simulink model "mirageTracking"  (R2015a)
settings: Solver=FixedStepDiscrete  StartTime=0.0  StopTime=10  FixedStep=1/30  RelTol=1e-3
undefined symbols (not defined in the file or in its folder): IsPositionTracked, IsSkeletonTracked, JointDepthIndices, JointImageIndices, JointTrackingState, JointWorldCoordinates, none, PositionDepthIndices, PositionImageIndices, PositionWorldCoordinates, SegmentationData, SkeletonTrackingID, videoinput
libraries: imaqlib x2
settings Model: xpc_rtwmakecfg_data=_jpeg_  CovSFcnEnable=off  Creator=sd0016  LastModifiedBy=sd0016
settings DebuggingCC: SolverPrmCheckMsg=warning
settings RTWCC: BuildConfiguration=Faster Runs

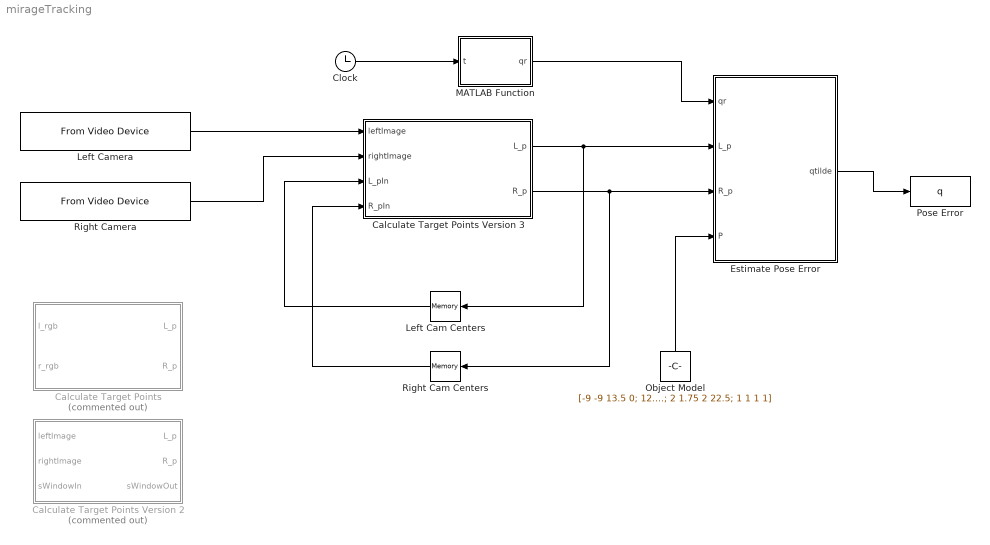
== system mirageTracking ==
  Calculate Target Points : MATLAB Function  Commented=on  TreatAsAtomicUnit=on
  Calculate Target Points Version 2 : MATLAB Function  Commented=on  TreatAsAtomicUnit=on
  Calculate Target Points Version 3 : MATLAB Function  TreatAsAtomicUnit=on
  Clock : Clock
  Estimate Pose Error : MATLAB Function  TreatAsAtomicUnit=on
  Left Cam Centers : Memory  X0=[598.500000000000,692.500000000000,645.500000000000,645.045454545455;681.157142857143,682.500000000000,673.159090909091,602.681818181818]  InheritSampleTime=on
  Left Camera : imaqlib/From Video Device  DeviceMenu=(none)  Device=winvideo 1 (Logitech HD Webcam C525)  ObjConstructor=videoinput('winvideo', 1)  VideoFormatMenu=(none)  VideoFormat=RGB24_1280x960  VideoSource=input1  ROIPosition=[0 0 960 1280]  EnableHWTrigger=off  TriggerConfiguration=none/none  SampleTime=1/30  OutputPortsMode=One multidimensional signal  DataType=single  CanDoHWTrigger=no  ReturnedColorSpace=rgb  BlockHandle=1921.0006  ROIWidth=1280  ROIHeight=960  ROIColumn=0  ROIRow=0  EngXMLPath=C:\Program Files\MATLAB\R2015a\toolbox\imaq\imaq\private  DevXMLPath=C:\MATLAB\SupportPackages\R2015a\osgenericvideointerface\toolbox\imaq\supportpackages\genericvideo\adaptor\win64  EngLibPath=C:\Program Files\MATLAB\R2015a\toolbox\imaq\imaqblks\imaqmex\win64  ColorSpace=rgb  BayerSensorAlignment=grbg  AllMetadata=IsPositionTracked;IsSkeletonTracked;JointDepthIndices;JointImageIndices;JointTrackingState;JointWorldCoordinates;PositionDepthIndices;PositionImageIndices;PositionWorldCoordinates;SegmentationData;SkeletonTrackingID
  MATLAB Function : MATLAB Function  TreatAsAtomicUnit=on
  Object Model : Constant  Value=[-9 -9 13.5 0; 12.75 -12.75 0 0; 2 1.75 2 22.5; 1 1 1 1]  VectorParams1D=off
  Pose Error : ToWorkspace  VariableName=q  SampleTime=-1
  Right Cam Centers : Memory  X0=[566.500000000000,660.814516129032,616.161764705882,612.663934426230;756.500000000000,756.250000000000,747.161764705882,676.614754098361]  InheritSampleTime=on
  Right Camera : imaqlib/From Video Device  DeviceMenu=(none)  Device=winvideo 2 (Logitech HD Webcam C525)  ObjConstructor=videoinput('winvideo', 2)  VideoFormatMenu=(none)  VideoFormat=RGB24_1280x960  VideoSource=input1  ROIPosition=[0 0 960 1280]  EnableHWTrigger=off  TriggerConfiguration=none/none  SampleTime=1/30  OutputPortsMode=One multidimensional signal  DataType=single  CanDoHWTrigger=no  ReturnedColorSpace=rgb  BlockHandle=1921.0006  ROIWidth=1280  ROIHeight=960  ROIColumn=0  ROIRow=0  EngXMLPath=C:\Program Files\MATLAB\R2015a\toolbox\imaq\imaq\private  DevXMLPath=C:\MATLAB\SupportPackages\R2015a\osgenericvideointerface\toolbox\imaq\supportpackages\genericvideo\adaptor\win64  EngLibPath=C:\Program Files\MATLAB\R2015a\toolbox\imaq\imaqblks\imaqmex\win64  ColorSpace=rgb  BayerSensorAlignment=grbg  AllMetadata=IsPositionTracked;IsSkeletonTracked;JointDepthIndices;JointImageIndices;JointTrackingState;JointWorldCoordinates;PositionDepthIndices;PositionImageIndices;PositionWorldCoordinates;SegmentationData;SkeletonTrackingID
  wires:
  Clock/1 -> MATLAB Function/1(t)
  MATLAB Function/1(qr) -> Estimate Pose Error/1(qr)
  Object Model/1 -> Estimate Pose Error/4(P)
  Estimate Pose Error/1(qtilde) -> Pose Error/1
  Left Camera/1 -> Calculate Target Points Version 3/1(leftImage)
  Right Camera/1 -> Calculate Target Points Version 3/2(rightImage)
  Calculate Target Points Version 3/1(L_p) -> Left Cam Centers/1, Estimate Pose Error/2(L_p)
  Calculate Target Points Version 3/2(R_p) -> Right Cam Centers/1, Estimate Pose Error/3(R_p)
  Left Cam Centers/1 -> Calculate Target Points Version 3/3(L_pIn)
  Right Cam Centers/1 -> Calculate Target Points Version 3/4(R_pIn)

== matlab function mirageTracking/Calculate Target Points ==
  data: l_rgb input; L_p output; r_rgb input; R_p output
function [L_p, R_p] = getCenter(l_rgb,r_rgb)

    %#codegen
    L_p=zeros(2,4);
    R_p=zeros(2,4);
    
    %input left image(l_rgb), right image(r_rgb), Pose target position 
    [m,n,c]=size(l_rgb);
    
    %define image variables for processing
    l_gray=zeros(m,n);      r_gray=zeros(m,n);
    l_rgb1=zeros(m,n,c);    r_rgb1=zeros(m,n,c);
    l_rgb2=zeros(m,n);      r_rgb2=zeros(m,n);

    l_bw=false(m,n);        r_bw=false(m,n);
    
    l_rgb1 = imcomplement(l_rgb);        % converts RGB to CMY color space 
    r_rgb1 = imcomplement(r_rgb);        % converts RGB to CMY color space 
    
    l_gray = 0.2989 * l_rgb1(:,:,1) + 0.5870 * l_rgb1(:,:,2) + 0.1140 * l_rgb1(:,:,3); % rgb2gray(rgb) ;convert rgb to grayscale 
    r_gray = 0.2989 * r_rgb1(:,:,1) + 0.5870 * r_rgb1(:,:,2) + 0.1140 * r_rgb1(:,:,3); % rgb2gray(rgb) ;convert rgb to grayscale
    
    l_rgb2 = l_rgb1(:,:,3)-l_gray;       % imsubtract(rgb1(:,:,3),gray)
    r_rgb2 = r_rgb1(:,:,3)-r_gray;       % imsubtract(rgb1(:,:,3),gray) 
        
%     l_rgb2 = medfilt2(l_rgb2);     % medfilt2(rgb2,[3 3]);
%     r_rgb2 = medfilt2(r_rgb2);     % medfilt2(rgb2,[3 3]);
%       
%     l_rgb2 = myMat2gray(l_rgb2);
%     r_rgb2 = myMat2gray(r_rgb2);
     
    l_bw = l_rgb2 > 0.2;
    r_bw = r_rgb2 > 0.2;

    %finds yellow regions in image using BlobAnalysis.
    hblob = vision.BlobAnalysis;

    [~,l_center,~] = step(hblob, l_bw); % get [x y] is a centroid of region
    [~,r_center,~] = step(hblob, r_bw); % get [x y] is a centroid of region
    
    %Send Left Camera Points
    ml = size(l_center,1);
    if ml > 4
        ml = 4;
    end
    
    for i=1:ml
        L_p(:,i)=l_center(i,:);
    end
    
    %Send Right Camera Points
    mr = size(r_center,1);
    if mr > 4
        mr = 4;
    end
    for i=1:mr
        R_p(:,i)=r_center(i,:);
    end
        
    L_p = orderPoints(L_p,m); 
    R_p = orderPoints(R_p,m);
        
    L_p(2,:) = m - L_p(2,:);
    R_p(2,:) = m - R_p(2,:);
end

% function imgOut = myMat2gray(imgIn)
%     %#codegen
%     imgIn = double(imgIn);
%     
%     minL = min(imgIn(:));
%     
%     imgTmp = (imgIn - minL);
%     
%     maxL = max(imgTmp(:));
%     
%     imgOut = imgTmp/maxL;
% end

== matlab function mirageTracking/MATLAB Function ==
  data: t input; qr output
function qr  = desired(t)
%#codegen

% qr = [xr yr thetar]^T (reference trajectory)
% ur = [vr omegar]^T (reference control input that generates the reference trajetory in ideal conditions)

% A = 1;
% xL = 10;
% vx = 1;

% % 
% % desired x and y 
% xr = vx*t;
% yr = A*sin(2*pi*xr/xL);
% 
% % desired x and y derivatives
% xrdot = vx;
% yrdot = A*(2*pi/xL)*cos(2*pi*xr/xL);
% 
% % desired theta
% thetar = atan2(yrdot,xrdot);
% 
% % desired second derivatives
% xrddot = 0;
% yrddot = -A*(2*pi/xL)^2*sin(2*pi*xr/xL);
% 
% % desired theta derivative
% thetardot = (yrddot - xrddot*tan(thetar))/(xrdot*(1+tan(thetar)^2));
% 
% 
% vr     = sqrt(xrdot^2+yrdot^2);
% omegar = thetardot;

%--------------------------------------------
% 
% xr = vx*t - 30;
% yr = A*sin(2*pi*xr/xL) + 2;
% 
% % desired x and y derivatives
% xrdot = vx;
% yrdot = A*(2*pi/xL)*cos(2*pi*xr/xL);
% 
% % desired theta
% thetar = atan2(yrdot,xrdot);
% 
% % desired second derivatives
% xrddot = 0;
% yrddot = -A*(2*pi/xL)^2*sin(2*pi*xr/xL);
% 
% % desired theta derivative
% thetardot = (yrddot - xrddot*tan(thetar))/(xrdot*(1+tan(thetar)^2));
% 
% vr     = sqrt(xrdot^2+yrdot^2);
% omegar = thetardot;

%--------------------------------------------
% yr = vx*t - 30;
% xr = A*sin(2*pi*yr/xL) + 2;
% 
% yrdot = vx;
% xrdot = A*(2*pi/xL)*cos(2*pi*xr/xL);
% 
% desired theta
% thetar = atan2(yrdot,xrdot);
% thetardot = 0;
% 
% vr     = sqrt(xrdot^2+yrdot^2);
% omegar = thetardot;

%--------------------------------------------
% xr = vx*t - 30;
% yr = 5;
% 
% xrdot = vx;
% yrdot = 0;
% 
% thetar = 0;
% thetardot = 0;
% 
% vr     = sqrt(xrdot^2+yrdot^2);
% omegar = thetardot;

% qr = [xr;yr;thetar];
% ur = [vr;omegar];

qr = [-395 2 45 0 0 0]';

== matlab function mirageTracking/Estimate Pose Error ==
  data: qr input; qtilde output; L_p input; R_p input; P input
function qtilde = mirage(qr,L_p,R_p,P)
%#codegen

%Desired Robot Pose for current step qr()
robotPoseDes.x = qr(1);
robotPoseDes.y = qr(2);
robotPoseDes.z = qr(3);
robotPoseDes.phi = qr(4);
robotPoseDes.theta = qr(5);
robotPoseDes.psi = qr(6);

%Transform target points from I space into Desired Robot Space
world2robotDes = inv(EulerTrans(robotPoseDes));
S_PDes = world2robotDes*P;

%Calculate the error parameters for current step
errParams = visioMotor(L_p,R_p,S_PDes);

poseErrorMat = eye(4,4);
poseErrorMat(1:3,:) = reshape(errParams,3,4);

world2robot = poseErrorMat*world2robotDes;

robotPoseEst = calculatePose(world2robot);

qtilde = [ -robotPoseEst.x  - robotPoseDes.x;
           -robotPoseEst.y  - robotPoseDes.y;
           -robotPoseEst.z  - robotPoseDes.z;
           -robotPoseEst.phi  - robotPoseDes.phi;
           -robotPoseEst.theta  - robotPoseDes.theta;
           -robotPoseEst.psi  - robotPoseDes.psi;];
       
end

== matlab function mirageTracking/Calculate Target Points Version 2 ==
  data: leftImage input; L_p output; rightImage input; sWindowIn input; R_p output; sWindowOut output
function [L_p, R_p, sWindowOut] = getCenterV2(leftImage, rightImage, sWindowIn)

    %#codegen
    L_p=zeros(2,4);
    R_p=zeros(2,4);
    
    m = size(leftImage,1);
    sWindowOut = zeros(8,4);
    
    for i=1:4
        lw = sWindowIn(i,:);
        lwx = (1:80) + lw(1);
        lwy = (1:80) + lw(2);
        
        rw = sWindowIn(i+4,:);
        rwx = (1:80) + rw(1);
        rwy = (1:80) + rw(2);
        
        pWinL = leftImage(lwy,lwx,:);
        pWinR = rightImage(rwy,rwx,:);
                
        pWinL = imcomplement(pWinL);        
        pWinR = imcomplement(pWinR);        
    
        pGrayL = 0.2989 * pWinL(:,:,1) + 0.5870 * pWinL(:,:,2) + 0.1140 * pWinL(:,:,3);
        pGrayR = 0.2989 * pWinR(:,:,1) + 0.5870 * pWinR(:,:,2) + 0.1140 * pWinR(:,:,3);
    
        pWinLF = pWinL(:,:,3)-pGrayL;       % imsubtract(rgb1(:,:,3),gray)
        pWinRF = pWinR(:,:,3)-pGrayR;       % imsubtract(rgb1(:,:,3),gray) 

        pBWL = pWinLF > 0.2;
        pBWR = pWinRF > 0.2;

        hblob = vision.BlobAnalysis; %finds yellow regions in image using BlobAnalysis.

        [~,cL,bbL] = step(hblob, pBWL); % get [x y] is a centroid of region
        [~,cR,bbR] = step(hblob, pBWR); % get [x y] is a centroid of region
        
        L_p(:,i) = cL(1,:) + lw(1:2);
        R_p(:,i) = cR(1,:) + rw(1:2);
        
        coeffL = double([-0.3 0;0 -0.3;0.3 0;0 0.3]); szL = double(bbL(1,3:4)');
        coeffR = double([-0.3 0;0 -0.3;0.3 0;0 0.3]); szR = double(bbR(1,3:4)');
        
        sWindowOut(i,:)   = round([lw(1); lw(2); 0; 0] + double(bbL(1,:)') + coeffL*szL)';
        sWindowOut(i+4,:) = round([rw(1); rw(2); 0; 0] + double(bbR(1,:)') + coeffR*szR)';
    end
    
    L_p(2,:) = m - L_p(2,:);
    R_p(2,:) = m - R_p(2,:);
end

== matlab function mirageTracking/Calculate Target Points Version 3 ==
  data: leftImage input; L_p output; rightImage input; L_pIn input; R_pIn input; R_p output
function [L_p, R_p] = getCenterV3(leftImage, rightImage, L_pIn, R_pIn)
    %#codegen 
    ps = 40; %Pad Size
    leftImage = padarray(leftImage,[ps ps],'both');
    rightImage = padarray(rightImage,[ps ps],'both');
    
    lwc = round(L_pIn) + ps; %Center of the left windows
    rwc = round(R_pIn) + ps; %Center of the right windows
    
    L_p = zeros(2,4);
    R_p = zeros(2,4);
    
    winRng = -40:40;
    for i=1:4
        lwx = winRng + lwc(1,i);
        lwy = winRng + lwc(2,i);
        
        rwx = winRng + rwc(1,i);
        rwy = winRng + rwc(2,i);
        
        pWinL = leftImage(lwy,lwx,:);
        pWinR = rightImage(rwy,rwx,:);
                
        pWinL = imcomplement(pWinL);        
        pWinR = imcomplement(pWinR);        
    
        pGrayL = 0.2989 * pWinL(:,:,1) + 0.5870 * pWinL(:,:,2) + 0.1140 * pWinL(:,:,3);
        pGrayR = 0.2989 * pWinR(:,:,1) + 0.5870 * pWinR(:,:,2) + 0.1140 * pWinR(:,:,3);
    
        pWinLF = pWinL(:,:,3)-pGrayL;       % imsubtract(rgb1(:,:,3),gray)
        pWinRF = pWinR(:,:,3)-pGrayR;       % imsubtract(rgb1(:,:,3),gray) 

        hautoth = vision.Autothresholder;
        pBWL = step(hautoth,pWinLF);
        pBWR = step(hautoth,pWinRF);

        %finds yellow regions in image using BlobAnalysis.
        hblob = vision.BlobAnalysis;

        [aL,cL,~] = step(hblob, pBWL); % get [x y] is a centroid of region
        [aR,cR,~] = step(hblob, pBWR); % get [x y] is a centroid of region
        
        [~, indL] = sort(aL,'descend');
        [~, indR] = sort(aR,'descend');
        
        L_p(:,i) = cL(indL(1),:)' + [lwx(1);lwy(1)] - [ps;ps];
        R_p(:,i) = cR(indR(1),:)' + [rwx(1);rwy(1)] - [ps;ps]; 
    end
end
